simulink model "gm_SignalGenerator"  (R2026a)
settings: Solver=VariableStepAuto  StartTime=0  StopTime=5e-5  MaxStep=5e-12  RelTol=1e-8
libraries: dsphdlxfrm2 x1, simulink x1
settings Model: Creator=adams  LastModifiedBy=adams
settings OptimizationCC: ConditionallyExecuteInputs=off
settings DebuggingCC: InheritedTsInSrcMsg=none
settings SimscapeCC: SimscapeLogType=none  SimscapeNominalValues="[{\"value\":\"1\",\"unit\":\"A\"},{\"value\":\"1\",\"unit\":\"bar\"},{\"value\":\"1\",\"unit\":\"cm^2\"},{\"value\":\"1\",\"unit\":\"cm^3/s\"},{\"value\":\"1\",\"unit\":\"kJ/kg\"},{\"value\":\"1\",\"unit\":\"kW\"},{\"value\":\"1\",\"unit\":\"l\"},{\"value\":\"1\",\"unit\":\"N\"},{\"value\":\"1\",\"unit\":\"N*m\"},{\"value\":\"1\",\"unit\":\"V\"}]"  SimscapeLogDataHistory=5000.0

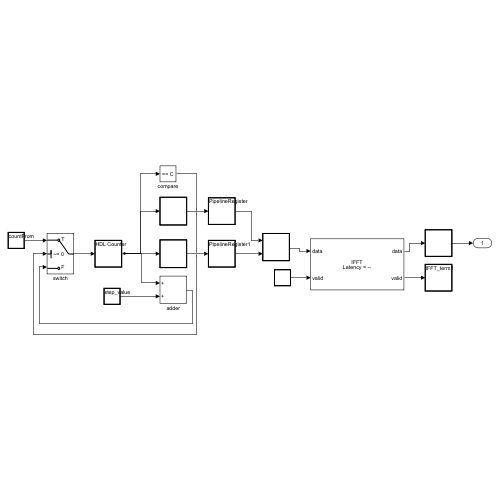
[thumbnail: Simulink's stored preview of the top-level diagram]
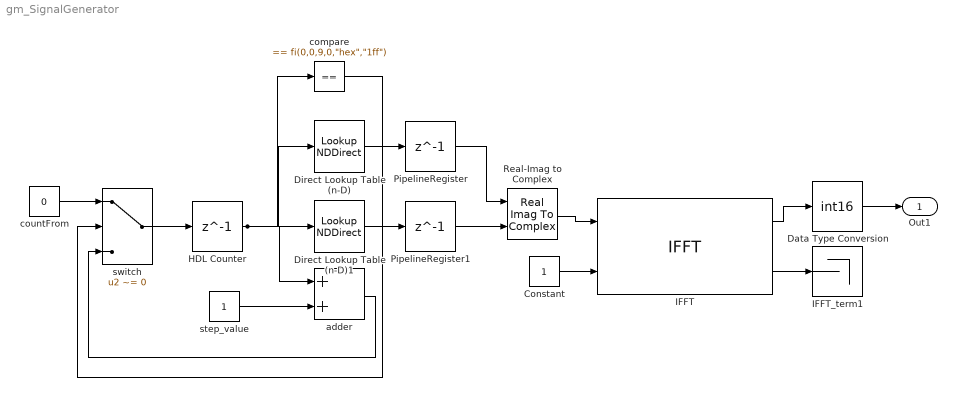
== system gm_SignalGenerator ==
  Constant : Constant  OutDataTypeStr=boolean  SampleTime=3.25520833333333e-09
  Data Type Conversion : DataTypeConversion  OutDataTypeStr=int16  RndMeth=Nearest  SampleTime=3.25520833333333e-09  SaturateOnIntegerOverflow=off
  Direct Lookup Table (n-D) : LookupNDDirect  NumberOfTableDimensions=1  Table="reshape(double([0;0;0;0;0;0;0;0;0;0;0;0;0;0;0;0;0;0;0;0;0;0;0;0;0;0;0;0;0;0;0;0;0;0;0;0;0;0;0;0;0;0;0;0;0;0;0;0;0;0;10000;0;0;0;0;0;0;0;0;0;0;0;0;0;0;0;0;0;0;0;0;0;0;0;0;0;0;0;0;0;0;0;0;0;0;0;0;0;0;0;0;0;0;0;0;0;0;0;0;0;0;0;0;0;0;0;0;0;0;0;0;0;0;0;0;0;0;0;0;0;0;0;0;0;0;0;0;0;0;0;0;0;0;0;0;0;0;0;0;0;0;0;0;0;0;0;0;0;0;0;0;0;0;0;0;0;0;0;0;0;0;0;0;0;0;0;0;0;0;0;0;0;0;0;0;0;0;0;0;0;0;0;0;0;0;0;0;0;0;0;0;0;0;0;0;0;0;0;0;0;0;0;0;0;0;0;0;0;0;0;0;0;0;0;0;0;0;0;0;0;0;0;0;0;0;0;0;0;0;0;0;0;0;0;0;0;0;0;0;0;0;0;0;0;0;0;0;0;0;0;0;0;0;0;0;0;0;0;0;0;0;0;0;0;0;0;0;0;0;0;0;0;0;0;0;0;0;0;0;0;0;0;0;0;0;0;0;0;0;0;0;0;0;0;0;0;0;0;0;0;0;0;0;0;0;0;0;0;0;0;0;0;0;0;0;0;0;0;0;0;0;0;0;0;0;0;0;0;0;0;0;0;0;0;0;0;0;0;0;0;0;0;0;0;0;0;0;0;0;0;0;0;0;0;0;0;0;0;0;0;0;0;0;0;0;0;0;0;0;0;0;0;0;0;0;0;0;0;0;0;0;0;0;0;0;0;0;0;0;0;0;0;0;0;0;0;0;0;0;0;0;0;0;0;0;0;0;0;0;0;0;0;0;0;0;0;0;0;0;0;0;0;0;0;0;0;0;0;0;0;0;0;0;0;0;0;0;0;0;0;0;0;0;0;0;0;0;0;0;0;0;0;0;0;0;0;0;0;0;0;0;0;10000;0;0;0;0;0;0;0;0;0;0;0;0;0;0;0;0;0;0;0;0;0;0;0;0;0;0;0;0;0;0;0;0;0;0;0;0;0;0;0;0;0;0;0;0;0;0;0;0;0]), [512    1])"  SampleTime=3.25520833333333e-09  TableDataTypeStr=fixdt(1,32,17)
  Direct Lookup Table (n-D)1 : LookupNDDirect  NumberOfTableDimensions=1  Table="reshape(double([0;0;0;0;0;0;0;0;0;0;0;0;0;0;0;0;0;0;0;0;0;0;0;0;0;0;0;0;0;0;0;0;0;0;0;0;0;0;0;0;0;0;0;0;0;0;0;0;0;0;0;0;0;0;0;0;0;0;0;0;0;0;0;0;0;0;0;0;0;0;0;0;0;0;0;0;0;0;0;0;0;0;0;0;0;0;0;0;0;0;0;0;0;0;0;0;0;0;0;0;0;0;0;0;0;0;0;0;0;0;0;0;0;0;0;0;0;0;0;0;0;0;0;0;0;0;0;0;0;0;0;0;0;0;0;0;0;0;0;0;0;0;0;0;0;0;0;0;0;0;0;0;0;0;0;0;0;0;0;0;0;0;0;0;0;0;0;0;0;0;0;0;0;0;0;0;0;0;0;0;0;0;0;0;0;0;0;0;0;0;0;0;0;0;0;0;0;0;0;0;0;0;0;0;0;0;0;0;0;0;0;0;0;0;0;0;0;0;0;0;0;0;0;0;0;0;0;0;0;0;0;0;0;0;0;0;0;0;0;0;0;0;0;0;0;0;0;0;0;0;0;0;0;0;0;0;0;0;0;0;0;0;0;0;0;0;0;0;0;0;0;0;0;0;0;0;0;0;0;0;0;0;0;0;0;0;0;0;0;0;0;0;0;0;0;0;0;0;0;0;0;0;0;0;0;0;0;0;0;0;0;0;0;0;0;0;0;0;0;0;0;0;0;0;0;0;0;0;0;0;0;0;0;0;0;0;0;0;0;0;0;0;0;0;0;0;0;0;0;0;0;0;0;0;0;0;0;0;0;0;0;0;0;0;0;0;0;0;0;0;0;0;0;0;0;0;0;0;0;0;0;0;0;0;0;0;0;0;0;0;0;0;0;0;0;0;0;0;0;0;0;0;0;0;0;0;0;0;0;0;0;0;0;0;0;0;0;0;0;0;0;0;0;0;0;0;0;0;0;0;0;0;0;0;0;0;0;0;0;0;0;0;0;0;0;0;0;0;0;0;0;0;0;0;0;0;0;0;0;0;0;0;0;0;0;0;0;0;0;0;0;0;0;0;0;0;0;0;0;0;0;0;0;0;0;0;0;0;0;0;0;0;0;0;0;0;0;0;0;0;0;0;0;0;0;0;0;0;0;0;0;0]), [512    1])"  SampleTime=3.25520833333333e-09  TableDataTypeStr=fixdt(1,32,17)
  HDL Counter : Delay  DelayLength=1  InitialCondition=0  SampleTime=3.25520833333333e-09
  IFFT : dsphdlxfrm2/IFFT  Architecture=Streaming Radix 2^2  FFTLengthSource=Property  FFTLength=512  FFTLengthMax=1024  ComplexMultiplication=Use 3 multipliers and 5 adders  BitReversedOutput=off  BitReversedInput=off  Normalize=off  SimulateUsing=Code generation  RoundingMethod=Nearest  ResetInputPort=off  StartOutputPort=off  EndOutputPort=off
  IFFT_term1 : Terminator
  PipelineRegister : Delay  DelayLength=1  InitialCondition=0  SampleTime=3.25520833333333e-09
  PipelineRegister1 : Delay  DelayLength=1  InitialCondition=0  SampleTime=3.25520833333333e-09
  Real-Imag to Complex : RealImagToComplex  ConstantPart="fi(0,1,32,17,\"hex\",\"00000000\")"  SampleTime=3.25520833333333e-09
  adder : Sum  OutDataTypeStr=fixdt(0, 9, 0)  AccumDataTypeStr=fixdt(0, 9, 0)  SampleTime=3.25520833333333e-09
  compare : simulink/Logic and Bit Operations/Compare To Constant  relop===  const="fi(0,0,9,0,\"hex\",\"1ff\")"  OutDataTypeStr=boolean
  countFrom : Constant  Value=0  VectorParams1D=off  OutDataTypeStr=fixdt(0, 9, 0)  SampleTime=3.25520833333333e-09
  step_value : Constant  VectorParams1D=off  OutDataTypeStr=fixdt(0, 9, 0)  SampleTime=3.25520833333333e-09
  switch : Switch  Criteria=u2 ~= 0  Threshold="fi(0,0,1,0,\"hex\",\"0\")"  OutDataTypeStr=fixdt(0, 9, 0)  SampleTime=3.25520833333333e-09  SaturateOnIntegerOverflow=off  InputSameDT=off
  Out1 : Outport  SampleTime=3.25520833333333e-09
  wires:
  countFrom/1 -> switch/1
  switch/1 -> HDL Counter/1
  adder/1 -> switch/3
  step_value/1 -> adder/2
  HDL Counter/1 -> Direct Lookup Table (n-D)1/1, Direct Lookup Table (n-D)/1, compare/1, adder/1
  Direct Lookup Table (n-D)1/1 -> PipelineRegister1/1
  compare/1 -> switch/2
  Direct Lookup Table (n-D)/1 -> PipelineRegister/1
  PipelineRegister/1 -> Real-Imag to Complex/1
  PipelineRegister1/1 -> Real-Imag to Complex/2
  Real-Imag to Complex/1 -> IFFT/1
  Constant/1 -> IFFT/2
  IFFT/1 -> Data Type Conversion/1
  IFFT/2 -> IFFT_term1/1
  Data Type Conversion/1 -> Out1/1
